simulink model "gyroboy_ext"  (R2019a)
settings: Solver=FixedStepAuto  StartTime=0.0  StopTime=inf  FixedStep=Ts  RelTol=1e-3  EnableMultiTasking=on
PreLoadFcn:
  | config
  | preload
  | HW=1;
InitFcn:
  | plant
  | control
undefined symbols (not defined in the file): A1, A2, B1, B2, C1, C2, D, D1, D2, DiscIntNeverNeededParam, fw, g, h, Jm, Jw, K, K_PWM, M, Psi0, R, Ts, W, X, Y, Z
libraries: sm_lib x16, nesl_utility x10, legoev3lib x9, simulink_extras x3, simulink x3, discretizing x1
settings Model: SimulationMode=external  ExtModeTrigDuration=20000  Creator=roslovetspv  LastModifiedBy=Pavel Roslovets
settings SolverCC: ZeroCrossAlgorithm=Adaptive  PositivePriorityOrder=on
settings OptimizationCC: MaxStackSize=64
settings DebuggingCC: ParameterTunabilityLossMsg=error  PregeneratedLibrarySubsystemCodeDiagnostic=none  ArithmeticOperatorsInVariantConditions=warning
settings HardwareCC: ProdBitPerPointer=32  ProdBitPerSizeT=32  ProdBitPerPtrDiffT=32  ProdLargestAtomicInteger=Long  ProdWordSize=32  ProdHWDeviceType=ARM Compatible->ARM 9
settings SFSimCC: SimUseLocalCustomCode=off  MATLABDynamicMemAlloc=off
settings RTWCC: SystemTargetFile=ert.tlc  HardwareBoard=LEGO MINDSTORMS EV3  TLCOptions="-aInlineSetEventsForThisBaseRateFcn=TLC_FALSE -aSuppressMultiTaskScheduler=TLC_FALSE  -aRateBasedStepFcn=0"  TemplateMakefile=ert_default_tmf  GenerateReport=on  RTWUseLocalCustomCode=off  Toolchain=Sourcery G++ Lite v2009q3  IncludeHyperlinkInReport=on  LaunchReport=on  GenerateTraceInfo=on  GenerateTraceReport=on  GenerateTraceReportSl=on  GenerateTraceReportSf=on  GenerateTraceReportEml=on
settings CodeAppCC: ForceParamTrailComments=on  IgnoreCustomStorageClasses=off  OperatorAnnotations=on  SimulinkDataObjDesc=on  SFDataObjDesc=on  MATLABFcnDesc=on  InsertBlockDesc=on  StateflowObjectComments=on  MATLABSourceComments=on
settings ERTTargetCC: MultiwordLength=2048  SupportContinuousTime=on  SupportVariableSizeSignals=on
settings ExplorerConfigSet: InternalSimMechanicsExplorerSettings="<ExplorerConfiguration><canonicalview>default</canonicalview><AnimationSetting><BasePlaybackSpeed>1.0</BasePlaybackSpeed><PlaybackSpeedFactor>1.0</PlaybackSpeedFactor></AnimationSetting><TilePanel><TileInfo><Tiles Columns=\"1\" Count=\"1\" Rows=\"1\"><Column Weight=\"1\"/><Row Weight=\"1\"/><Tile Height=\"1\" Width=\"1\" X=\"0\" Y=\"0\"/></Tiles></TileInfo><SceneInfo><SceneViewer><BGColor><R>1</R><G>1</G><B>1</B></BGColor><Camera><DoPerspective>off</DoPerspective><Position><X>0.737677845990044934</X><Y>-0.67856704951033231</Y><Z>0.394310698325195552</Z></Position><Center><X>0.13835347465754938</X><Y>0.0549599908195436276</Y><Z>0.0737668182840573866</Z></Center><Up><X>-0.28491224059991338</X><Y>0.178745032231141465</Y><Z>0.941740531467678998</Z></Up><ViewLimDist>1</ViewLimDist><YLim>0.238341914277370809</YLim><XLim>0.445475675236847168</XLim></Camera></SceneViewer></SceneInfo></TilePanel><MechEditorPanel><Cameras/><GfxPanelCameraMap/><VideoCreator><PlaybackSpeedRatio>1.0</PlaybackSpeedRatio><FrameRate>30</FrameRate><VideoFormat>Motion JPEG AVI</VideoFormat><FrameSize>auto</FrameSize></VideoCreator></MechEditorPanel></ExplorerConfiguration>"

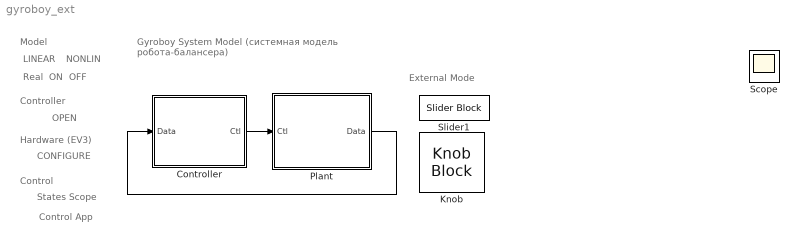
== system gyroboy_ext ==
  note: External Mode
  note: Control
  note: States Scope
  note: OPEN
  note: Controller
  note: Hardware (EV3)
  note: Model
  note: Real
  note: Gyroboy System Model
      | (системная модель робота-балансера)
  note: ON
  note: OFF
  note: CONFIGURE
  note: LINEAR
  note: NONLIN
  note: Control App
  Controller : Subsystem
      mask Display: image('img/brain.png')
  Knob : KnobBlock  ScaleMin=-10  ScaleMax=10  TickInterval=1
  Plant : Subsystem  Variant=on  VariantControl=Variant1
      mask Display:
      | if evalin('base','HW')
      |     image('img/gyroboy.png')
      | elseif evalin('base','MB')
      |     image('img/multibody.png')
      | else
      |     image('img/math.png')
      | end
  Slider1 : SliderBlock  ScaleMin=-10  ScaleMax=10  TickInterval=1
  Scope : Scope
  wires:
  Controller/1(Ctl) -> Plant/1("Ctl ")
  Plant/1(" Data") -> Controller/1(Data)

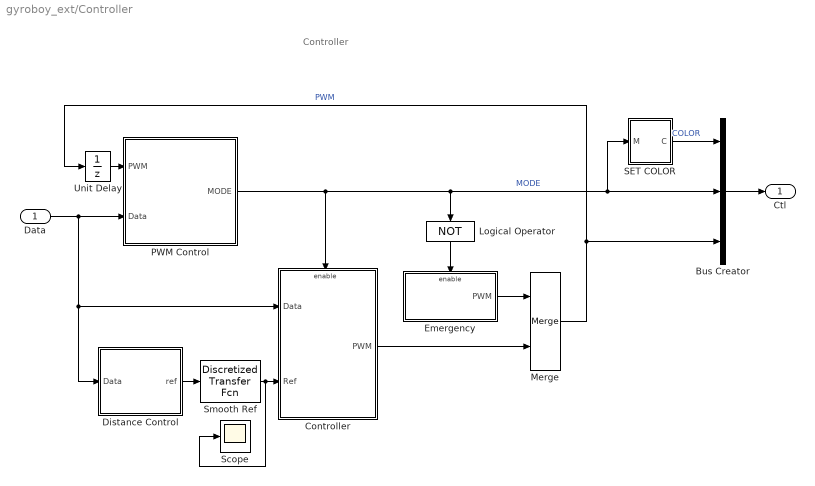
== system gyroboy_ext/Controller ==
  note: Controller
  Data : Inport
  Bus Creator : BusCreator  Inputs=3
  Controller : Subsystem  TreatAsAtomicUnit=on
      mask Display: disp('ON')
  Distance Control : Stateflow chart  TreatAsAtomicUnit=on
  Emergency : Subsystem  TreatAsAtomicUnit=on
      mask Display: disp('OFF')
  Logical Operator : Logic  Operator=NOT  AllPortsSameDT=off  OutDataTypeStr=boolean
  Merge : Merge
  PWM Control : Stateflow chart  TreatAsAtomicUnit=on
  SET COLOR : MATLAB Function  TreatAsAtomicUnit=on
  Scope : Scope
  Smooth Ref : discretizing/Discretized Transfer Fcn  Numerator=[1]  Denominator=[0.7 1]  AbsTol=auto  SampleTime=Ts  method=zoh  Wc=1
      settings: SourceProductName=Simulink  SourceProductBaseCode=SL
  Unit Delay : UnitDelay  SampleTime=-1  HasFrameUpgradeWarning=on
  Ctl : Outport
  wires:
  Merge/1 -> Unit Delay/1, Bus Creator/3  "PWM"
  PWM Control/1(MODE) -> Logical Operator/1, Bus Creator/2, SET COLOR/1(M), Controller/Enable  "MODE"
  Data/1 -> PWM Control/2(Data), Distance Control/1(Data), Controller/1(Data)
  Controller/1(PWM) -> Merge/2
  Emergency/1(PWM) -> Merge/1
  Unit Delay/1 -> PWM Control/1(PWM)
  Logical Operator/1 -> Emergency/Enable
  Bus Creator/1 -> Ctl/1
  SET COLOR/1(C) -> Bus Creator/1  "COLOR"
  Distance Control/1(ref) -> Smooth Ref/1
  Smooth Ref/1 -> Scope/1, Controller/2(Ref)

== system gyroboy_ext/Plant ==
  "Ctl " : Inport
  EV3 : Subsystem  VariantControl=HW==1
  Model : Subsystem  VariantControl=(default)
  " Data" : Outport

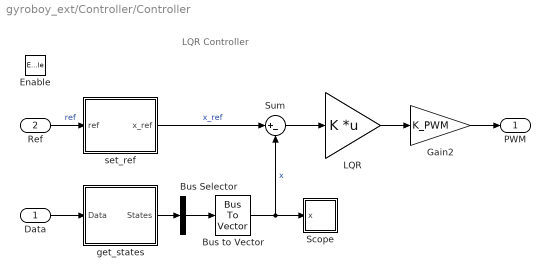
== system gyroboy_ext/Controller/Controller ==
  note: LQR Controller
  Data : Inport
  Ref : Inport  Port=2
  Enable : EnablePort  StatesWhenEnabling=reset
  Bus Selector : BusSelector  OutputSignals=theta_int,theta,psi,theta_dot,psi_dot,phi,phi_dot  OutputAsBus=on
  Bus to Vector : BusToVector
  Gain2 : Gain  Gain=K_PWM
  LQR : Gain  Gain=K  Multiplication=Matrix(K*u)
  Scope : Subsystem
  Sum : Sum  Inputs=|+-
  get_states : Subsystem
  set_ref : Subsystem
  PWM : Outport
  wires:
  Data/1 -> get_states/1(Data)
  Sum/1 -> LQR/1
  Bus Selector/1 -> Bus to Vector/1
  get_states/1(States) -> Bus Selector/1
  LQR/1 -> Gain2/1
  Bus to Vector/1 -> Sum/2, Scope/1(x)  "x"
  Ref/1 -> set_ref/1(ref)  "ref"
  Gain2/1 -> PWM/1
  set_ref/1(x_ref) -> Sum/1  "x_ref"

== system gyroboy_ext/Controller/Distance Control/Normal ==
  Data : Inport  OutDataTypeStr=Bus: Data
  Action Port : ActionPort
      settings: CopyFcn=Stateflow.SLINSF.SimulinkMan.removeBlockPreDeleteFcn  PreDeleteFcn=Stateflow.SLINSF.SimulinkMan.unsafePredeleteFcn
  Bus Selector2 : BusSelector  OutputSignals=udp
  Demux : Demux  Outputs=2
  Gain : Gain  Gain=0.75
  Gain1 : Gain  Gain=0.2
  Mux : Mux  Inputs=2
  ref : Outport  PortDimensions=2
  wires:
  Gain1/1 -> Mux/2
  Mux/1 -> ref/1  "ref"
  Gain/1 -> Mux/1
  Demux/1 -> Gain/1  "Vel"
  Demux/2 -> Gain1/1  "Turn"
  Data/1 -> Bus Selector2/1
  Bus Selector2/1 -> Demux/1  "<udp>"

== system gyroboy_ext/Controller/Distance Control/STOP ==
  Data : Inport  OutDataTypeStr=Bus: Data
  Action Port : ActionPort
      settings: CopyFcn=Stateflow.SLINSF.SimulinkMan.removeBlockPreDeleteFcn  PreDeleteFcn=Stateflow.SLINSF.SimulinkMan.unsafePredeleteFcn
  Constant : Constant  Value=[0 0]
  Terminator : Terminator
  ref : Outport  PortDimensions=2
  wires:
  Data/1 -> Terminator/1
  Constant/1 -> ref/1

== system gyroboy_ext/Controller/Emergency ==
  Enable : EnablePort  StatesWhenEnabling=reset
  Constant : Constant  Value=[0 0]
  PWM : Outport
  wires:
  Constant/1 -> PWM/1

== system gyroboy_ext/Controller/PWM Control/On.check ==
  PWM : Inport  OutDataTypeStr=double  PortDimensions=2
  f : TriggerPort  TriggerType=function-call  VariantControl=(inherit)
      settings: CopyFcn=Stateflow.SLINSF.SimulinkMan.removeBlockPreDeleteFcn  PreDeleteFcn=Stateflow.SLINSF.SimulinkMan.unsafePredeleteFcn
  Abs : Abs
  Compare To Constant : simulink/Logic and Bit Operations/Compare To Constant  relop=<  const=200  OutDataTypeStr=boolean
  Sum of Elements : Sum  Inputs=+
  OK : Outport  PortDimensions=1
  wires:
  PWM/1 -> Abs/1
  Abs/1 -> Sum of Elements/1
  Sum of Elements/1 -> Compare To Constant/1
  Compare To Constant/1 -> OK/1

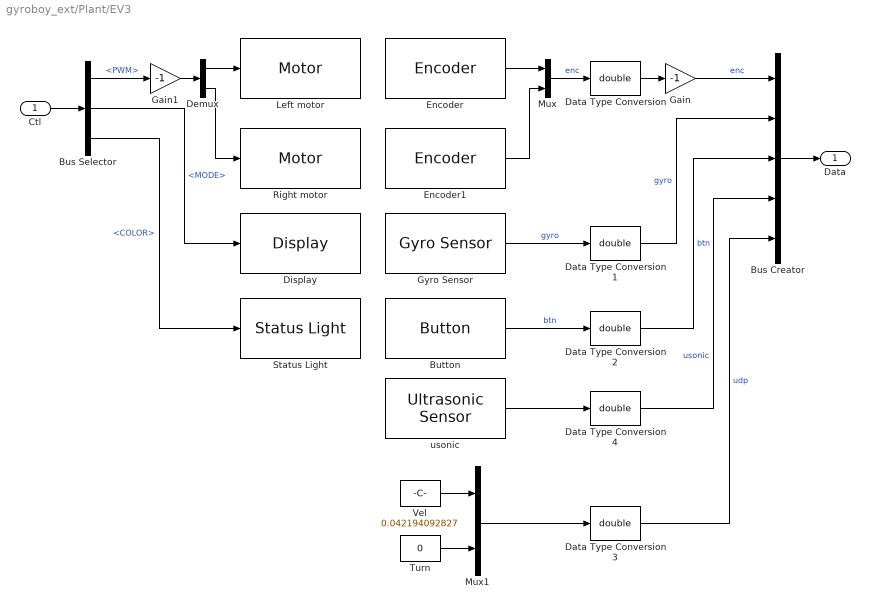
== system gyroboy_ext/Plant/EV3 ==
  Ctl : Inport
  Bus Creator : BusCreator  Inputs=5
  Bus Selector : BusSelector  OutputSignals=PWM,MODE,COLOR
  Button : legoev3lib/Button  buttonType=Up  sampleTime=Ts
      settings: SourceProductName=Simulink Support Package for LEGO MINDSTORMS EV3 Hardware  SourceProductBaseCode=LEGOEV3
  Data Type Conversion{,1..4} (5 alike) : DataTypeConversion  OutDataTypeStr=double
  Demux : Demux  Outputs=2
  Display : legoev3lib/Display  slcdStr=RUNNING  slcdLine=1  slcdFormat=Decimal
      settings: SourceProductName=Simulink Support Package for LEGO MINDSTORMS EV3 Hardware  SourceProductBaseCode=LEGOEV3
  Encoder : legoev3lib/Encoder  portNumber=D  opMode=No reset  sampleTime=Ts
      settings: SourceProductName=Simulink Support Package for LEGO MINDSTORMS EV3 Hardware  SourceProductBaseCode=LEGOEV3
  Encoder1 : legoev3lib/Encoder  portNumber=A  opMode=No reset  sampleTime=Ts
      settings: SourceProductName=Simulink Support Package for LEGO MINDSTORMS EV3 Hardware  SourceProductBaseCode=LEGOEV3
  Gain : Gain  Gain=-1
  Gain1 : Gain  Gain=-1
  Gyro Sensor : legoev3lib/Gyro Sensor  portNumber=2  sampleTime=Ts
      settings: SourceProductName=Simulink Support Package for LEGO MINDSTORMS EV3 Hardware  SourceProductBaseCode=LEGOEV3
  Left motor : legoev3lib/Motor  sportNumber=D  sstopAction=Brake
  Mux : Mux  Inputs=2
  Mux1 : Mux  Inputs=2
  Right motor : legoev3lib/Motor  sportNumber=A  sstopAction=Brake
  Status Light : legoev3lib/Status Light
      settings: SourceProductName=Simulink Support Package for LEGO MINDSTORMS EV3 Hardware  SourceProductBaseCode=LEGOEV3
  Turn : Constant  Value=0
  Vel : Constant  Value=0.042194092827
  usonic : legoev3lib/Ultrasonic Sensor  PortNumber=4  sampleTime=Ts
      settings: SourceProductName=Simulink Support Package for LEGO MINDSTORMS EV3 Hardware  SourceProductBaseCode=LEGOEV3
  Data : Outport
  wires:
  Ctl/1 -> Bus Selector/1
  Encoder/1 -> Mux/1
  Encoder1/1 -> Mux/2
  Gyro Sensor/1 -> Data Type Conversion1/1  "gyro"
  Bus Selector/1 -> Gain1/1  "<PWM>"
  Mux/1 -> Data Type Conversion/1  "enc"
  Bus Creator/1 -> Data/1
  Demux/1 -> Left motor/1
  Demux/2 -> Right motor/1
  Data Type Conversion/1 -> Gain/1
  Data Type Conversion1/1 -> Bus Creator/2  "gyro"
  Gain/1 -> Bus Creator/1  "enc"
  Gain1/1 -> Demux/1
  Bus Selector/2 -> Display/1  "<MODE>"
  Button/1 -> Data Type Conversion2/1  "btn"
  Data Type Conversion2/1 -> Bus Creator/3  "btn"
  Bus Selector/3 -> Status Light/1  "<COLOR>"
  Data Type Conversion3/1 -> Bus Creator/5  "udp"
  usonic/1 -> Data Type Conversion4/1
  Data Type Conversion4/1 -> Bus Creator/4  "usonic"
  Vel/1 -> Mux1/1
  Turn/1 -> Mux1/2
  Mux1/1 -> Data Type Conversion3/1

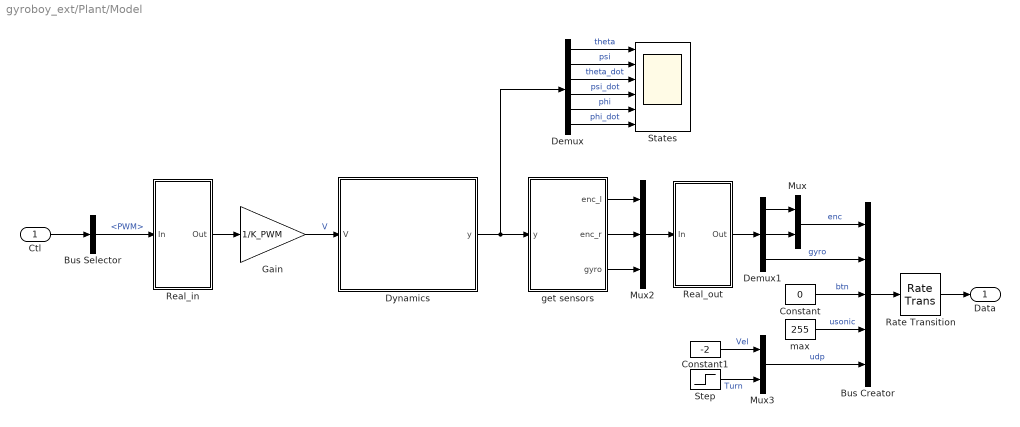
== system gyroboy_ext/Plant/Model ==
  Ctl : Inport
  Bus Creator : BusCreator  Inputs=5
  Bus Selector : BusSelector  OutputSignals=PWM
  Constant : Constant  Value=0
  Constant1 : Constant  Value=-2
  Demux : Demux  Outputs=6
  Demux1 : Demux  Outputs=3
  Dynamics : Subsystem  Variant=on  VariantControl=Variant1
  Gain : Gain  Gain=1/K_PWM
  Mux : Mux  Inputs=2
  Mux2 : Mux  Inputs=3
  Mux3 : Mux  Inputs=2
  Rate Transition : RateTransition  OutPortSampleTime=Ts
  Real_in : Subsystem  Variant=on  VariantControl=Variant1
  Real_out : Subsystem  Variant=on  VariantControl=Variant1
  States : Scope  NumInputPorts=6
  Step : Step  Time=3  Before=1  After=0  SampleTime=0
  get sensors : MATLAB Function  TreatAsAtomicUnit=on
  max : Constant  Value=255
  Data : Outport
  wires:
  Real_in/1(" Out") -> Gain/1
  Ctl/1 -> Bus Selector/1
  Mux2/1 -> Real_out/1("In ")
  get sensors/3(gyro) -> Mux2/3
  Real_out/1(" Out") -> Demux1/1
  Demux/4 -> States/4  "psi_dot"
  Demux/6 -> States/6  "phi_dot"
  Demux/5 -> States/5  "phi"
  Bus Creator/1 -> Rate Transition/1
  Demux1/1 -> Mux/1
  Demux1/2 -> Mux/2
  Demux1/3 -> Bus Creator/2  "gyro"
  Demux/2 -> States/2  "psi"
  Demux/3 -> States/3  "theta_dot"
  Demux/1 -> States/1  "theta"
  Bus Selector/1 -> Real_in/1(In)  "<PWM>"
  get sensors/1(enc_l) -> Mux2/1
  get sensors/2(enc_r) -> Mux2/2
  Mux/1 -> Bus Creator/1  "enc"
  Rate Transition/1 -> Data/1
  Constant/1 -> Bus Creator/3  "btn"
  Constant1/1 -> Mux3/1  "Vel"
  Step/1 -> Mux3/2  "Turn"
  Mux3/1 -> Bus Creator/5  "udp"
  Gain/1 -> Dynamics/1("V ")  "V"
  Dynamics/1(" y") -> Demux/1, get sensors/1(y)
  max/1 -> Bus Creator/4  "usonic"

== system gyroboy_ext/Controller/Controller/Scope ==
  x : Inport
  Demux : Demux  Outputs=7
  Scope : Scope  NumInputPorts=7
  wires:
  Demux/7 -> Scope/7  "phi_dot"
  Demux/5 -> Scope/5  "psi_dot"
  Demux/3 -> Scope/3  "psi"
  Demux/6 -> Scope/6  "phi"
  Demux/2 -> Scope/2  "theta"
  Demux/1 -> Scope/1  "theta_int"
  Demux/4 -> Scope/4  "theta_dot"
  x/1 -> Demux/1

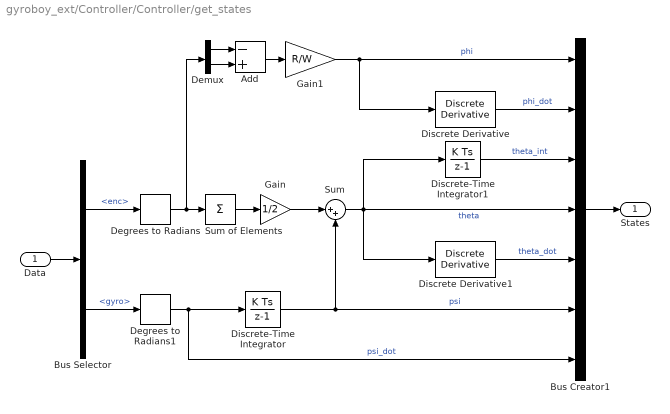
== system gyroboy_ext/Controller/Controller/get_states ==
  Data : Inport
  Add : Sum  Inputs=-+
  Bus Creator1 : BusCreator  Inputs=7
  Bus Selector : BusSelector  OutputSignals=enc,gyro
  Degrees to Radians : simulink_extras/Transformations/Degrees to Radians
  Degrees to Radians1 : simulink_extras/Transformations/Degrees to Radians
  Demux : Demux  Outputs=2
  Discrete Derivative : simulink/Discrete/Discrete Derivative  gainval=1.0  ICPrevScaledInput=0.0  OutMin=[]  OutMax=[]  OutDataType=fixdt(1, 16)  OutScaling=2^-10  DoSatur=off
  Discrete Derivative1 : simulink/Discrete/Discrete Derivative  gainval=1.0  ICPrevScaledInput=0.0  OutMin=[]  OutMax=[]  OutDataType=fixdt(1, 16)  OutScaling=2^-10  DoSatur=off
  Discrete-Time Integrator : DiscreteIntegrator  SampleTime=-1  ICPrevOutput=DiscIntNeverNeededParam  ICPrevScaledInput=DiscIntNeverNeededParam
  Discrete-Time Integrator1 : DiscreteIntegrator  SampleTime=-1  ICPrevOutput=DiscIntNeverNeededParam  ICPrevScaledInput=DiscIntNeverNeededParam
  Gain : Gain  Gain=1/2
  Gain1 : Gain  Gain=R/W
  Sum : Sum  Inputs=|++
  Sum of Elements : Sum  Inputs=+
  States : Outport
  wires:
  Gain/1 -> Sum/1
  Degrees to Radians/1 -> Demux/1, Sum of Elements/1
  Data/1 -> Bus Selector/1
  Bus Selector/1 -> Degrees to Radians/1  "<enc>"
  Sum/1 -> Discrete-Time Integrator1/1, Discrete Derivative1/1, Bus Creator1/4  "theta"
  Bus Creator1/1 -> States/1
  Sum of Elements/1 -> Gain/1
  Degrees to Radians1/1 -> Discrete-Time Integrator/1, Bus Creator1/7  "psi_dot"
  Bus Selector/2 -> Degrees to Radians1/1  "<gyro>"
  Demux/1 -> Add/1
  Demux/2 -> Add/2
  Add/1 -> Gain1/1
  Gain1/1 -> Discrete Derivative/1, Bus Creator1/1  "phi"
  Discrete Derivative/1 -> Bus Creator1/2  "phi_dot"
  Discrete Derivative1/1 -> Bus Creator1/5  "theta_dot"
  Discrete-Time Integrator/1 -> Sum/2, Bus Creator1/6  "psi"
  Discrete-Time Integrator1/1 -> Bus Creator1/3  "theta_int"

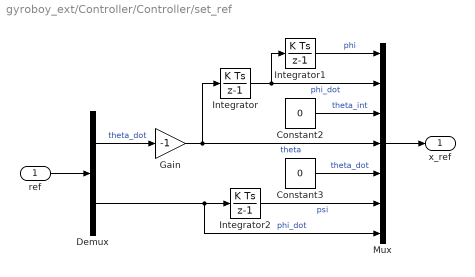
== system gyroboy_ext/Controller/Controller/set_ref ==
  ref : Inport
  Constant2 : Constant  Value=0
  Constant3 : Constant  Value=0
  Demux : Demux  Outputs=2
  Gain : Gain  Gain=-1
  Integrator : DiscreteIntegrator  SampleTime=Ts  ICPrevOutput=DiscIntNeverNeededParam  ICPrevScaledInput=DiscIntNeverNeededParam  mask(DiscretizedDiscreteIntegrator){}
      mask init:
      | %zoh
  Integrator1 : DiscreteIntegrator  SampleTime=Ts  ICPrevOutput=DiscIntNeverNeededParam  ICPrevScaledInput=DiscIntNeverNeededParam  mask(DiscretizedDiscreteIntegrator){}
      mask init:
      | %zoh
  Integrator2 : DiscreteIntegrator  SampleTime=Ts  ICPrevOutput=DiscIntNeverNeededParam  ICPrevScaledInput=DiscIntNeverNeededParam  mask(DiscretizedDiscreteIntegrator){}
      mask init:
      | %zoh
  Mux : Mux  Inputs=7
  x_ref : Outport
  wires:
  Constant2/1 -> Mux/3  "theta_int"
  Constant3/1 -> Mux/5  "theta_dot"
  Mux/1 -> x_ref/1
  Integrator/1 -> Mux/2, Integrator1/1  "phi_dot"
  Demux/2 -> Mux/7, Integrator2/1  "phi_dot"
  Integrator2/1 -> Mux/6  "psi"
  Integrator1/1 -> Mux/1  "phi"
  Demux/1 -> Gain/1  "theta_dot"
  ref/1 -> Demux/1
  Gain/1 -> Integrator/1, Mux/4  "theta"

== system gyroboy_ext/Plant/Model/Dynamics ==
  "V " : Inport
  Multibody (nonlinear) : Subsystem  VariantControl=MB == 1
  State-space (linear) : Subsystem  VariantControl=(default)
  " y" : Outport

== system gyroboy_ext/Plant/Model/Real_in ==
  In : Inport
  Ideal_in : Subsystem  VariantControl=(default)
  Real_in : Subsystem  VariantControl=real_model == 1
  " Out" : Outport

== system gyroboy_ext/Plant/Model/Real_out ==
  "In " : Inport
  Ideal_out : Subsystem  VariantControl=(default)
  Real_out : Subsystem  VariantControl=real_model == 1
  " Out" : Outport

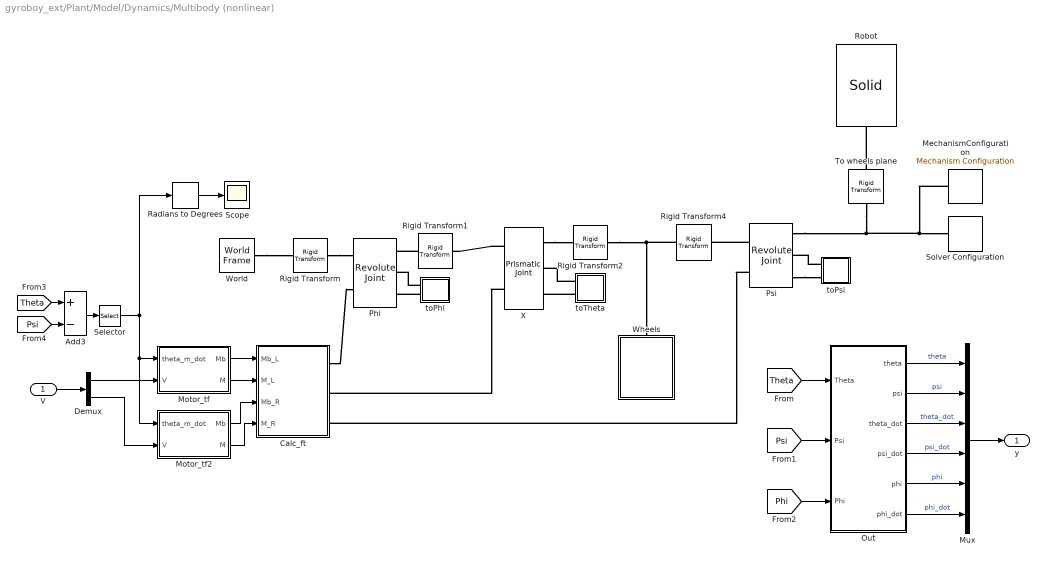
== system gyroboy_ext/Plant/Model/Dynamics/Multibody (nonlinear) ==
  V : Inport
  Add3 : Sum  Inputs=+-
  Calc_ft : Subsystem
  Demux : Demux  Outputs=2
  MechanismConfiguration : sm_lib/Utilities/Mechanism Configuration  UniformGravity=Constant  GravityVector=[0 0 -g]  GravityUnits=m/s^2  LinearizationDelta=0.00001
  Motor_tf : Subsystem  mask{Kt=0.0209, Rm=1, b=0.0113, Km=0, Tm=0}
  Motor_tf2 : Subsystem  mask{Kt=0.0209, Rm=1, b=0.0113, Km=0, Tm=0}
  Mux : Mux  Inputs=6
  Out : Subsystem
  Phi : sm_lib/Joints/Revolute Joint  SenseConstraintForce=off  SenseConstraintForceX=off  SenseConstraintForceY=off  SenseConstraintForceZ=off  SenseConstraintTorque=off  SenseConstraintTorqueX=off  SenseConstraintTorqueY=off  SenseConstraintTorqueZ=off  SenseTotalForce=off  SenseTotalForceX=off  SenseTotalForceY=off  SenseTotalForceZ=off  SenseTotalTorque=off  SenseTotalTorqueX=off  SenseTotalTorqueY=off  SenseTotalTorqueZ=off  CompositeWrenchDir=FollowerOnBase  CompositeWrenchFrame=BaseFrame  EquilibriumPosition=0  EquilibriumPositionUnits=deg  SpringStiffness=0  SpringStiffnessUnits=N*m/deg  DampingCoefficient=W^2/R^2/2*(0.0113+fw)  DampingCoefficientUnits=N*m/(rad/s)  TorqueActuationMode=InputTorque  MotionActuationMode=ComputedMotion  SensePosition=on  SenseVelocity=on  SenseAcceleration=off  SenseTorqueForce=off  SenseLowerLimitTorqueForce=off  SenseUpperLimitTorqueForce=off  LowerLimitSpecify=off  LowerLimitBound=-90  LowerLimitBoundUnits=deg  LowerLimitStiffness=1e4  LowerLimitStiffnessUnits=N*m/deg  LowerLimitDamping=10  LowerLimitDampingUnits=N*m/(deg/s)  LowerLimitTransitionRegionWidth=0.1  LowerLimitTransitionRegionWidthUnits=deg  UpperLimitSpecify=off  UpperLimitBound=90  UpperLimitBoundUnits=deg  UpperLimitStiffness=1e4  UpperLimitStiffnessUnits=N*m/deg  UpperLimitDamping=10  UpperLimitDampingUnits=N*m/(deg/s)  UpperLimitTransitionRegionWidth=0.1  UpperLimitTransitionRegionWidthUnits=deg  PositionTargetSpecify=off  PositionTargetPriority=High  PositionTargetValue=0  PositionTargetValueUnits=deg  VelocityTargetSpecify=off  VelocityTargetPriority=High  VelocityTargetValue=0  VelocityTargetValueUnits=deg/s
  Psi : sm_lib/Joints/Revolute Joint  SenseConstraintForce=off  SenseConstraintForceX=off  SenseConstraintForceY=off  SenseConstraintForceZ=off  SenseConstraintTorque=off  SenseConstraintTorqueX=off  SenseConstraintTorqueY=off  SenseConstraintTorqueZ=off  SenseTotalForce=off  SenseTotalForceX=off  SenseTotalForceY=off  SenseTotalForceZ=off  SenseTotalTorque=off  SenseTotalTorqueX=off  SenseTotalTorqueY=off  SenseTotalTorqueZ=off  CompositeWrenchDir=FollowerOnBase  CompositeWrenchFrame=BaseFrame  EquilibriumPosition=0  EquilibriumPositionUnits=deg  SpringStiffness=0  SpringStiffnessUnits=N*m/deg  DampingCoefficient=0  DampingCoefficientUnits=N*m/(deg/s)  TorqueActuationMode=InputTorque  MotionActuationMode=ComputedMotion  SensePosition=on  SenseVelocity=on  SenseAcceleration=off  SenseTorqueForce=off  SenseLowerLimitTorqueForce=off  SenseUpperLimitTorqueForce=off  LowerLimitSpecify=off  LowerLimitBound=-90  LowerLimitBoundUnits=deg  LowerLimitStiffness=1e4  LowerLimitStiffnessUnits=N*m/deg  LowerLimitDamping=10  LowerLimitDampingUnits=N*m/(deg/s)  LowerLimitTransitionRegionWidth=0.1  LowerLimitTransitionRegionWidthUnits=deg  UpperLimitSpecify=off  UpperLimitBound=90  UpperLimitBoundUnits=deg  UpperLimitStiffness=1e4  UpperLimitStiffnessUnits=N*m/deg  UpperLimitDamping=10  UpperLimitDampingUnits=N*m/(deg/s)  UpperLimitTransitionRegionWidth=0.1  UpperLimitTransitionRegionWidthUnits=deg  PositionTargetSpecify=on  PositionTargetPriority=High  PositionTargetValue=Psi0  PositionTargetValueUnits=rad  VelocityTargetSpecify=off  VelocityTargetPriority=High  VelocityTargetValue=1  VelocityTargetValueUnits=deg/s
  Radians to Degrees : simulink_extras/Transformations/Radians to Degrees
  Rigid Transform : sm_lib/Frames and Transforms/Rigid Transform  TranslationMethod=Cartesian  TranslationStandardOffset=0  TranslationLengthUnit=m  TranslationStandardAxis=+Z  TranslationCartesianOffset=[0 0 R]  TranslationROffset=0  TranslationROffsetUnits=m  TranslationZOffset=0  TranslationZOffsetUnits=m  TranslationThetaOffset=0  TranslationThetaOffsetUnits=deg  RotationMethod=None  RotationAngleUnits=deg  RotationStandardAxis=+Z  RotationAngle=0.0  RotationArbitraryAxis=[0 0 1]  FollAlignAxisA=+X  BaseAlignAxisA=+Y  FollAlignAxisB=+Y  BaseAlignAxisB=+Z  RotationSequenceAxes=FollowerAxes  RotationSequence=XYX  RotationSequenceAngles=[0 0 0]  RotationSequenceAnglesUnits=deg  RotationMatrix=[1 0 0; 0 1 0; 0 0 1]
  Rigid Transform1 : sm_lib/Frames and Transforms/Rigid Transform  TranslationMethod=None  TranslationStandardOffset=0  TranslationLengthUnit=m  TranslationStandardAxis=+Z  TranslationCartesianOffset=[0 0 0]  TranslationROffset=0  TranslationROffsetUnits=m  TranslationZOffset=0  TranslationZOffsetUnits=m  TranslationThetaOffset=0  TranslationThetaOffsetUnits=deg  RotationMethod=StandardAxis  RotationAngleUnits=deg  RotationStandardAxis=+Y  RotationAngle=90  RotationArbitraryAxis=[0 0 1]  FollAlignAxisA=+X  BaseAlignAxisA=+Y  FollAlignAxisB=+Y  BaseAlignAxisB=+Z  RotationSequenceAxes=FollowerAxes  RotationSequence=XYX  RotationSequenceAngles=[0 0 0]  RotationSequenceAnglesUnits=deg  RotationMatrix=[1 0 0; 0 1 0; 0 0 1]
  Rigid Transform2 : sm_lib/Frames and Transforms/Rigid Transform  TranslationMethod=None  TranslationStandardOffset=0  TranslationLengthUnit=m  TranslationStandardAxis=+Z  TranslationCartesianOffset=[0 0 0]  TranslationROffset=0  TranslationROffsetUnits=m  TranslationZOffset=0  TranslationZOffsetUnits=m  TranslationThetaOffset=0  TranslationThetaOffsetUnits=deg  RotationMethod=StandardAxis  RotationAngleUnits=deg  RotationStandardAxis=+Y  RotationAngle=90  RotationArbitraryAxis=[0 0 1]  FollAlignAxisA=+X  BaseAlignAxisA=+Y  FollAlignAxisB=+Y  BaseAlignAxisB=+Z  RotationSequenceAxes=FollowerAxes  RotationSequence=XYX  RotationSequenceAngles=[0 0 0]  RotationSequenceAnglesUnits=deg  RotationMatrix=[1 0 0; 0 1 0; 0 0 1]
  Rigid Transform4 : sm_lib/Frames and Transforms/Rigid Transform  TranslationMethod=None  TranslationStandardOffset=0  TranslationLengthUnit=m  TranslationStandardAxis=+Z  TranslationCartesianOffset=[0 -W/2 0]  TranslationROffset=0  TranslationROffsetUnits=m  TranslationZOffset=0  TranslationZOffsetUnits=m  TranslationThetaOffset=0  TranslationThetaOffsetUnits=deg  RotationMethod=StandardAxis  RotationAngleUnits=deg  RotationStandardAxis=-X  RotationAngle=90  RotationArbitraryAxis=[0 0 1]  FollAlignAxisA=+X  BaseAlignAxisA=+Y  FollAlignAxisB=+Y  BaseAlignAxisB=+Z  RotationSequenceAxes=FollowerAxes  RotationSequence=XYX  RotationSequenceAngles=[0 0 0]  RotationSequenceAnglesUnits=deg  RotationMatrix=[1 0 0; 0 1 0; 0 0 1]
  Robot : sm_lib/Body Elements/Solid  InertiaType=CalculateFromGeometry  Mass=M  MassUnits=kg  CenterOfMass=[0 0 0]  CenterOfMassUnits=m  MomentsOfInertia=[1 1 1]  MomentsOfInertiaUnits=kg*m^2  ProductsOfInertia=[0 0 0]  ProductsOfInertiaUnits=kg*m^2  BasedOnType=Mass  Density=1000  DensityUnits=kg/(m^3)  DoExposeReferenceFrame=on  SerializedFrames=<Frames/>  GraphicType=FromGeometry  MarkerShape=Sphere  MarkerSize=10  GraphicVisPropType=SimpleVisualProperties  GraphicDiffuseColor=[0.0 1.0 0.4]  GraphicSpecularColor=[0.5 0.5 0.5 1.0]  GraphicAmbientColor=[0.15 0.15 0.15 1.0]  GraphicEmissiveColor=[0.0 0.0 0.0 1.0]  GraphicShininess=75  GraphicOpacity=1.0  GeometryShape=Brick  RectangleSize=[1 1]  RectangleSizeUnits=m  BrickDimensions=[D h W]  BrickDimensionUnits=m  CylinderRadius=1  CylinderRadiusUnits=m  CylinderLength=1  CylinderLengthUnits=m  SphereRadius=1  SphereRadiusUnits=m  EllipsoidRadii=[1 1 1]  EllipsoidRadiiUnits=m  ExtrusionCrossSection=[1 1; -1 1; -1 -1; 1 -1]  ExtrusionCrossSectionUnits=m  ExtrusionLength=1  ExtrusionLengthUnits=m  PolygonNumSides=3  PolygonOuterRadius=1  PolygonOuterRadiusUnits=m  ExtGeomFileType=STEP  ExtGeomFileUnits=m  RevolutionCrossSection=[1 1; 1 -1; 2 -1; 2 1]  RevolutionCrossSectionUnits=m  RevolutionExtent=Full  RevolutionAngle=180  RevolutionAngleUnits=deg
  Scope : Scope
  Selector : Selector  InputPortWidth=2  IndexOptions=Index vector (dialog)  Indices=2  OutputSizes=1
  Solver Configuration : nesl_utility/Solver Configuration  PhysicalDomain=network_engine_domain  SubClassName=solver  LeftPortType=input  RightPortType=generic  Tones=[]  Harmonics=[]  SimulateNoise=off  Profile=off  UseLocalSampling=off  EnableSwitchedLinearOptims=on  FrequencyDomain=off  UseCCode=off  RelTol=0.001  AbsTol=1e-06  MinStep=1e-09  ToWorkspace=off  RevertToSquareIcSolve=off  NumHomotopyIterations=100  PhasorMode=off  PhasorModeNumHarmonics=1  DoDC=off  ResidualTolerance=1e-09  UseLocalSolver=off  LocalSolverChoice=NE_TRAPEZOIDAL_ADVANCER  LocalSolverSampleTime=0.001  DoFixedCost=off  MaxNonlinIter=3  MaxModeIter=2  LinearAlgebra=Sparse  EquationFormulation=NE_TIME_EF  DelaysMemoryBudget=1024  AutomaticFiltering=on  FilteringTimeConstant=1e-6  PartitionStorageMethod=AS_NEEDED  PartitionMemoryBudget=1024  PartitionMethod=FAST
  To wheels plane : sm_lib/Frames and Transforms/Rigid Transform  TranslationMethod=Cartesian  TranslationStandardOffset=0  TranslationLengthUnit=m  TranslationStandardAxis=+Z  TranslationCartesianOffset=[0 h/2 0]  TranslationROffset=0  TranslationROffsetUnits=m  TranslationZOffset=0  TranslationZOffsetUnits=m  TranslationThetaOffset=0  TranslationThetaOffsetUnits=deg  RotationMethod=None  RotationAngleUnits=deg  RotationStandardAxis=+Z  RotationAngle=0.0  RotationArbitraryAxis=[0 0 1]  FollAlignAxisA=+X  BaseAlignAxisA=+Y  FollAlignAxisB=+Y  BaseAlignAxisB=+Z  RotationSequenceAxes=FollowerAxes  RotationSequence=XYX  RotationSequenceAngles=[0 0 0]  RotationSequenceAnglesUnits=deg  RotationMatrix=[1 0 0; 0 1 0; 0 0 1]
  Wheels : Subsystem
      mask Display:
      | plot(sin(0:0.01:10), cos(0:0.01:10))
      | plot(.5+sin(0:0.01:10), .5+cos(0:0.01:10))
  World : sm_lib/Frames and Transforms/World Frame
  X : sm_lib/Joints/Prismatic Joint  SenseConstraintForce=off  SenseConstraintForceX=off  SenseConstraintForceY=off  SenseConstraintForceZ=off  SenseConstraintTorque=off  SenseConstraintTorqueX=off  SenseConstraintTorqueY=off  SenseConstraintTorqueZ=off  SenseTotalForce=off  SenseTotalForceX=off  SenseTotalForceY=off  SenseTotalForceZ=off  SenseTotalTorque=off  SenseTotalTorqueX=off  SenseTotalTorqueY=off  SenseTotalTorqueZ=off  CompositeWrenchDir=FollowerOnBase  CompositeWrenchFrame=BaseFrame  EquilibriumPosition=0  EquilibriumPositionUnits=m  SpringStiffness=0  SpringStiffnessUnits=N/m  DampingCoefficient=0  DampingCoefficientUnits=N/(m/s)  TorqueActuationMode=InputTorque  MotionActuationMode=ComputedMotion  SensePosition=on  SenseVelocity=on  SenseAcceleration=off  SenseTorqueForce=off  SenseLowerLimitTorqueForce=off  SenseUpperLimitTorqueForce=off  LowerLimitSpecify=off  LowerLimitBound=-1  LowerLimitBoundUnits=m  LowerLimitStiffness=1e6  LowerLimitStiffnessUnits=N/m  LowerLimitDamping=1e3  LowerLimitDampingUnits=N/(m/s)  LowerLimitTransitionRegionWidth=1e-4  LowerLimitTransitionRegionWidthUnits=m  UpperLimitSpecify=off  UpperLimitBound=1  UpperLimitBoundUnits=m  UpperLimitStiffness=1e6  UpperLimitStiffnessUnits=N/m  UpperLimitDamping=1e3  UpperLimitDampingUnits=N/(m/s)  UpperLimitTransitionRegionWidth=1e-4  UpperLimitTransitionRegionWidthUnits=m  PositionTargetSpecify=off  PositionTargetPriority=High  PositionTargetValue=0  PositionTargetValueUnits=m  VelocityTargetSpecify=off  VelocityTargetPriority=High  VelocityTargetValue=0  VelocityTargetValueUnits=m/s
  toPhi : Subsystem
  toPsi : Subsystem
  toTheta : Subsystem
  y : Outport
  wires:
  [Theta] -> Out/1(Theta)
  [Psi] -> Out/2(Psi)
  Out/1(theta) -> Mux/1  "theta"
  Out/2(psi) -> Mux/2  "psi"
  Out/3(theta_dot) -> Mux/3  "theta_dot"
  Out/4(psi_dot) -> Mux/4  "psi_dot"
  Out/5(phi) -> Mux/5  "phi"
  Out/6(phi_dot) -> Mux/6  "phi_dot"
  [Phi] -> Out/3(Phi)
  Demux/1 -> Motor_tf/2(V)
  Demux/2 -> Motor_tf2/2(V)
  V/1 -> Demux/1
  Motor_tf/2(M) -> Calc_ft/2(M_L)
  Add3/1 -> Selector/1
  [Theta] -> Add3/1
  [Psi] -> Add3/2
  Motor_tf/1(Mb) -> Calc_ft/1(Mb_L)
  Motor_tf2/1(Mb) -> Calc_ft/3(Mb_R)
  Motor_tf2/2(M) -> Calc_ft/4(M_R)
  Selector/1 -> Motor_tf/1(theta_m_dot), Motor_tf2/1(theta_m_dot), Radians to Degrees/1
  Radians to Degrees/1 -> Scope/1
  Mux/1 -> y/1
  connections:
  MechanismConfiguration/RConn1 -- Solver Configuration/RConn1 -- Psi/RConn1 -- To wheels plane/RConn1
  Rigid Transform2/LConn1 -- Wheels/LConn1 -- Rigid Transform4/LConn1
  Rigid Transform/RConn1 -- Phi/LConn1
  World/RConn1 -- Rigid Transform/LConn1
  toTheta/LConn1 -- X/RConn2
  toPhi/LConn2 -- Phi/RConn3
  toPhi/LConn1 -- Phi/RConn2
  toTheta/LConn2 -- X/RConn3
  Calc_ft/RConn1 -- Phi/LConn2
  Psi/LConn2 -- Calc_ft/RConn3
  X/LConn1 -- Rigid Transform1/RConn1
  Rigid Transform1/LConn1 -- Phi/RConn1
  Psi/RConn3 -- toPsi/LConn2
  Psi/LConn1 -- Rigid Transform4/RConn1
  X/RConn1 -- Rigid Transform2/RConn1
  X/LConn2 -- Calc_ft/RConn2
  toPsi/LConn1 -- Psi/RConn2
  To wheels plane/LConn1 -- Robot/RConn1

== system gyroboy_ext/Plant/Model/Dynamics/State-space (linear) ==
  V : Inport
  Model1 : StateSpace  A=A1  B=B1  C=C1  D=D1  InitialCondition=[0 Psi0 0 0]
  Model2 : StateSpace  A=A2  B=B2  C=C2  D=D2  InitialCondition=0
  Mux1 : Mux  Inputs=2
  y : Outport
  wires:
  Model2/1 -> Mux1/2  "y2"
  Model1/1 -> Mux1/1  "y1"
  Mux1/1 -> y/1  "y"
  V/1 -> Model2/1, Model1/1

== system gyroboy_ext/Plant/Model/Real_in/Ideal_in ==
  In : Inport
  " Out" : Outport
  wires:
  In/1 -> " Out"/1

== system gyroboy_ext/Plant/Model/Real_in/Real_in ==
  In : Inport
  Rounding Function : Rounding  Operator=round
  Saturation : Saturate  UpperLimit=100  LowerLimit=-100
  " Out" : Outport
  wires:
  In/1 -> Rounding Function/1
  Saturation/1 -> " Out"/1
  Rounding Function/1 -> Saturation/1

== system gyroboy_ext/Plant/Model/Real_out/Ideal_out ==
  "In " : Inport
  " Out" : Outport
  wires:
  "In "/1 -> " Out"/1

== system gyroboy_ext/Plant/Model/Real_out/Real_out ==
  "In " : Inport
  Rounding Function : Rounding  Operator=round
  " Out" : Outport
  wires:
  "In "/1 -> Rounding Function/1
  Rounding Function/1 -> " Out"/1

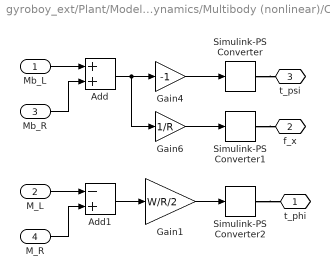
== system gyroboy_ext/Plant/Model/Dynamics/Multibody (nonlinear)/Calc_ft ==
  Mb_L : Inport
  M_L : Inport  Port=2
  Mb_R : Inport  Port=3
  M_R : Inport  Port=4
  Add : Sum
  Add1 : Sum  Inputs=-+
  Gain1 : Gain  Gain=W/R/2
  Gain4 : Gain  Gain=-1
  Gain6 : Gain  Gain=1/R
  Simulink-PS Converter : nesl_utility/Simulink-PS Converter  PhysicalDomain=network_engine_domain  SubClassName=ps_input  LeftPortType=input  RightPortType=output  PseudoPeriodic=off  Frequencies=[]  NoiseDistribution=none  NoiseParameters=[]  Unit=N*m  AffineConversion=off  FilteringAndDerivatives=zero  SimscapeFilterOrder=1  InputFilterTimeConstant=0.001  UdotUserProvided=1
  Simulink-PS Converter1 : nesl_utility/Simulink-PS Converter  PhysicalDomain=network_engine_domain  SubClassName=ps_input  LeftPortType=input  RightPortType=output  PseudoPeriodic=off  Frequencies=[]  NoiseDistribution=none  NoiseParameters=[]  Unit=N  AffineConversion=off  FilteringAndDerivatives=zero  SimscapeFilterOrder=1  InputFilterTimeConstant=0.001  UdotUserProvided=1
  Simulink-PS Converter2 : nesl_utility/Simulink-PS Converter  PhysicalDomain=network_engine_domain  SubClassName=ps_input  LeftPortType=input  RightPortType=output  PseudoPeriodic=off  Frequencies=[]  NoiseDistribution=none  NoiseParameters=[]  Unit=N*m  AffineConversion=off  FilteringAndDerivatives=zero  SimscapeFilterOrder=1  InputFilterTimeConstant=0.001  UdotUserProvided=1
  t_phi : PMIOPort  Side=Right
  f_x : PMIOPort  Port=2  Side=Right
  t_psi : PMIOPort  Port=3  Side=Right
  wires:
  Add/1 -> Gain6/1, Gain4/1
  Mb_L/1 -> Add/1
  M_L/1 -> Add1/1
  Add1/1 -> Gain1/1
  Mb_R/1 -> Add/2
  M_R/1 -> Add1/2
  Gain4/1 -> Simulink-PS Converter/1
  Gain6/1 -> Simulink-PS Converter1/1
  Gain1/1 -> Simulink-PS Converter2/1
  connections:
  Simulink-PS Converter2/RConn1 -- t_phi/RConn1
  Simulink-PS Converter/RConn1 -- t_psi/RConn1
  Simulink-PS Converter1/RConn1 -- f_x/RConn1

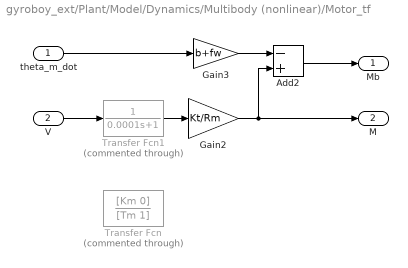
== system gyroboy_ext/Plant/Model/Dynamics/Multibody (nonlinear)/Motor_tf ==
  theta_m_dot : Inport
  V : Inport  Port=2
  Add2 : Sum  Inputs=-+
  Gain2 : Gain  Gain=Kt/Rm
  Gain3 : Gain  Gain=b+fw
  Transfer Fcn : TransferFcn  Commented=through  Numerator=[Km 0]  Denominator=[Tm 1]
  Transfer Fcn1 : TransferFcn  Commented=through  Denominator=[0.0001 1]
  Mb : Outport
  M : Outport  Port=2
  wires:
  Transfer Fcn1/1 -> Gain2/1
  Add2/1 -> Mb/1
  Gain3/1 -> Add2/1
  theta_m_dot/1 -> Gain3/1
  Gain2/1 -> M/1, Add2/2
  V/1 -> Transfer Fcn1/1

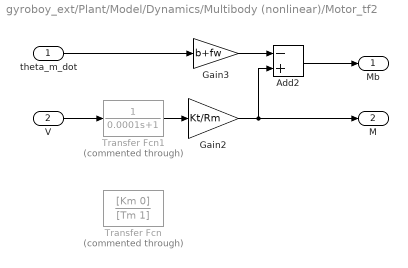
== system gyroboy_ext/Plant/Model/Dynamics/Multibody (nonlinear)/Motor_tf2 ==
  theta_m_dot : Inport
  V : Inport  Port=2
  Add2 : Sum  Inputs=-+
  Gain2 : Gain  Gain=Kt/Rm
  Gain3 : Gain  Gain=b+fw
  Transfer Fcn : TransferFcn  Commented=through  Numerator=[Km 0]  Denominator=[Tm 1]
  Transfer Fcn1 : TransferFcn  Commented=through  Denominator=[0.0001 1]
  Mb : Outport
  M : Outport  Port=2
  wires:
  Transfer Fcn1/1 -> Gain2/1
  Add2/1 -> Mb/1
  Gain3/1 -> Add2/1
  theta_m_dot/1 -> Gain3/1
  Gain2/1 -> M/1, Add2/2
  V/1 -> Transfer Fcn1/1

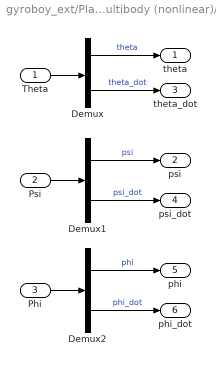
== system gyroboy_ext/Plant/Model/Dynamics/Multibody (nonlinear)/Out ==
  Theta : Inport
  Psi : Inport  Port=2
  Phi : Inport  Port=3
  Demux : Demux  Outputs=2
  Demux1 : Demux  Outputs=2
  Demux2 : Demux  Outputs=2
  theta : Outport
  psi : Outport  Port=2
  theta_dot : Outport  Port=3
  psi_dot : Outport  Port=4
  phi : Outport  Port=5
  phi_dot : Outport  Port=6
  wires:
  Psi/1 -> Demux1/1
  Theta/1 -> Demux/1
  Demux1/1 -> psi/1  "psi"
  Demux/1 -> theta/1  "theta"
  Demux1/2 -> psi_dot/1  "psi_dot"
  Demux/2 -> theta_dot/1  "theta_dot"
  Demux2/1 -> phi/1  "phi"
  Demux2/2 -> phi_dot/1  "phi_dot"
  Phi/1 -> Demux2/1

== system gyroboy_ext/Plant/Model/Dynamics/Multibody (nonlinear)/Wheels ==
  Base : sm_lib/Body Elements/Solid  InertiaType=CalculateFromGeometry  Mass=(Jw+Jm)/R^2*2  MassUnits=kg  CenterOfMass=[0 0 0]  CenterOfMassUnits=m  MomentsOfInertia=[1 1 1]  MomentsOfInertiaUnits=kg*m^2  ProductsOfInertia=[0 0 0]  ProductsOfInertiaUnits=kg*m^2  BasedOnType=Mass  Density=1000  DensityUnits=kg/(m^3)  DoExposeReferenceFrame=on  SerializedFrames=<Frames/>  GraphicType=None  MarkerShape=Sphere  MarkerSize=10  GraphicVisPropType=SimpleVisualProperties  GraphicDiffuseColor=[0.5 0.5 0.5]  GraphicSpecularColor=[0.5 0.5 0.5 1.0]  GraphicAmbientColor=[0.15 0.15 0.15 1.0]  GraphicEmissiveColor=[0.0 0.0 0.0 1.0]  GraphicShininess=75  GraphicOpacity=1.0  GeometryShape=Brick  RectangleSize=[1 1]  RectangleSizeUnits=m  BrickDimensions=[1 1 .5]*0.1  BrickDimensionUnits=m  CylinderRadius=1  CylinderRadiusUnits=m  CylinderLength=1  CylinderLengthUnits=m  SphereRadius=1  SphereRadiusUnits=m  EllipsoidRadii=[1 1 1]  EllipsoidRadiiUnits=m  ExtrusionCrossSection=[1 1; -1 1; -1 -1; 1 -1]  ExtrusionCrossSectionUnits=m  ExtrusionLength=1  ExtrusionLengthUnits=m  PolygonNumSides=3  PolygonOuterRadius=1  PolygonOuterRadiusUnits=m  ExtGeomFileType=STEP  ExtGeomFileUnits=m  RevolutionCrossSection=[1 1; 1 -1; 2 -1; 2 1]  RevolutionCrossSectionUnits=m  RevolutionExtent=Full  RevolutionAngle=180  RevolutionAngleUnits=deg
  Rigid Transform1 : sm_lib/Frames and Transforms/Rigid Transform  TranslationMethod=StandardAxis  TranslationStandardOffset=0.05  TranslationLengthUnit=m  TranslationStandardAxis=-Y  TranslationCartesianOffset=[0 0 0]  TranslationROffset=0  TranslationROffsetUnits=m  TranslationZOffset=0  TranslationZOffsetUnits=m  TranslationThetaOffset=0  TranslationThetaOffsetUnits=deg  RotationMethod=StandardAxis  RotationAngleUnits=deg  RotationStandardAxis=+X  RotationAngle=90  RotationArbitraryAxis=[0 0 1]  FollAlignAxisA=+X  BaseAlignAxisA=+Y  FollAlignAxisB=+Y  BaseAlignAxisB=+Z  RotationSequenceAxes=FollowerAxes  RotationSequence=XYX  RotationSequenceAngles=[0 0 0]  RotationSequenceAnglesUnits=deg  RotationMatrix=[1 0 0; 0 1 0; 0 0 1]
  Rigid Transform3 : sm_lib/Frames and Transforms/Rigid Transform  TranslationMethod=StandardAxis  TranslationStandardOffset=0.05  TranslationLengthUnit=m  TranslationStandardAxis=+Y  TranslationCartesianOffset=[0 0 0]  TranslationROffset=0  TranslationROffsetUnits=m  TranslationZOffset=0  TranslationZOffsetUnits=m  TranslationThetaOffset=0  TranslationThetaOffsetUnits=deg  RotationMethod=StandardAxis  RotationAngleUnits=deg  RotationStandardAxis=+X  RotationAngle=90  RotationArbitraryAxis=[0 0 1]  FollAlignAxisA=+X  BaseAlignAxisA=+Y  FollAlignAxisB=+Y  BaseAlignAxisB=+Z  RotationSequenceAxes=FollowerAxes  RotationSequence=XYX  RotationSequenceAngles=[0 0 0]  RotationSequenceAnglesUnits=deg  RotationMatrix=[1 0 0; 0 1 0; 0 0 1]
  Wheel1 : sm_lib/Body Elements/Solid  InertiaType=PointMass  Mass=0  MassUnits=g  CenterOfMass=[0 0 0]  CenterOfMassUnits=m  MomentsOfInertia=[0 0 0]  MomentsOfInertiaUnits=kg*m^2  ProductsOfInertia=[0 0 0]  ProductsOfInertiaUnits=kg*m^2  BasedOnType=Mass  Density=1000  DensityUnits=kg/(m^3)  DoExposeReferenceFrame=on  SerializedFrames=<Frames/>  GraphicType=FromGeometry  MarkerShape=Sphere  MarkerSize=10  GraphicVisPropType=SimpleVisualProperties  GraphicDiffuseColor=[1.0 0.4 0.4]  GraphicSpecularColor=[0.5 0.5 0.5 1.0]  GraphicAmbientColor=[0.15 0.15 0.15 1.0]  GraphicEmissiveColor=[0.0 0.0 0.0 1.0]  GraphicShininess=75  GraphicOpacity=1.0  GeometryShape=Cylinder  RectangleSize=[1 1]  RectangleSizeUnits=m  BrickDimensions=[1 1 1]  BrickDimensionUnits=m  CylinderRadius=R  CylinderRadiusUnits=m  CylinderLength=0.02  CylinderLengthUnits=m  SphereRadius=1  SphereRadiusUnits=m  EllipsoidRadii=[1 1 1]  EllipsoidRadiiUnits=m  ExtrusionCrossSection=[1 1; -1 1; -1 -1; 1 -1]  ExtrusionCrossSectionUnits=m  ExtrusionLength=1  ExtrusionLengthUnits=m  PolygonNumSides=3  PolygonOuterRadius=1  PolygonOuterRadiusUnits=m  ExtGeomFileType=STEP  ExtGeomFileUnits=m  RevolutionCrossSection=[1 1; 1 -1; 2 -1; 2 1]  RevolutionCrossSectionUnits=m  RevolutionExtent=Full  RevolutionAngle=180  RevolutionAngleUnits=deg
  Wheel2 : sm_lib/Body Elements/Solid  InertiaType=PointMass  Mass=0  MassUnits=g  CenterOfMass=[0 0 0]  CenterOfMassUnits=m  MomentsOfInertia=[0 0 0]  MomentsOfInertiaUnits=kg*m^2  ProductsOfInertia=[0 0 0]  ProductsOfInertiaUnits=kg*m^2  BasedOnType=Mass  Density=1000  DensityUnits=kg/(m^3)  DoExposeReferenceFrame=on  SerializedFrames=<Frames/>  GraphicType=FromGeometry  MarkerShape=Sphere  MarkerSize=10  GraphicVisPropType=SimpleVisualProperties  GraphicDiffuseColor=[1.0 0.4 0.4]  GraphicSpecularColor=[0.5 0.5 0.5 1.0]  GraphicAmbientColor=[0.15 0.15 0.15 1.0]  GraphicEmissiveColor=[0.0 0.0 0.0 1.0]  GraphicShininess=75  GraphicOpacity=1.0  GeometryShape=Cylinder  RectangleSize=[1 1]  RectangleSizeUnits=m  BrickDimensions=[1 1 1]  BrickDimensionUnits=m  CylinderRadius=R  CylinderRadiusUnits=m  CylinderLength=0.02  CylinderLengthUnits=m  SphereRadius=1  SphereRadiusUnits=m  EllipsoidRadii=[1 1 1]  EllipsoidRadiiUnits=m  ExtrusionCrossSection=[1 1; -1 1; -1 -1; 1 -1]  ExtrusionCrossSectionUnits=m  ExtrusionLength=1  ExtrusionLengthUnits=m  PolygonNumSides=3  PolygonOuterRadius=1  PolygonOuterRadiusUnits=m  ExtGeomFileType=STEP  ExtGeomFileUnits=m  RevolutionCrossSection=[1 1; 1 -1; 2 -1; 2 1]  RevolutionCrossSectionUnits=m  RevolutionExtent=Full  RevolutionAngle=180  RevolutionAngleUnits=deg
  B : PMIOPort  Side=Left
  connections:
  Wheel2/RConn1 -- Rigid Transform3/RConn1
  Wheel1/RConn1 -- Rigid Transform1/RConn1
  Rigid Transform1/LConn1 -- Base/RConn1 -- Rigid Transform3/LConn1 -- B/RConn1

== system gyroboy_ext/Plant/Model/Dynamics/Multibody (nonlinear)/toPhi ==
  Mux : Mux  Inputs=2
  PS-Simulink Converter : nesl_utility/PS-Simulink Converter  PhysicalDomain=network_engine_domain  SubClassName=ps_output  LeftPortType=input  RightPortType=output  PseudoPeriodic=off  Frequencies=[]  Unit=rad  AffineConversion=off
  PS-Simulink Converter1 : nesl_utility/PS-Simulink Converter  PhysicalDomain=network_engine_domain  SubClassName=ps_output  LeftPortType=input  RightPortType=output  PseudoPeriodic=off  Frequencies=[]  Unit=rad/s  AffineConversion=off
  q : PMIOPort  Side=Left
  w : PMIOPort  Port=2  Side=Left
  tag scope: Phi=global
  wires:
  PS-Simulink Converter/1 -> Mux/1
  PS-Simulink Converter1/1 -> Mux/2
  Mux/1 -> [Phi]
  connections:
  PS-Simulink Converter/LConn1 -- q/RConn1
  PS-Simulink Converter1/LConn1 -- w/RConn1

== system gyroboy_ext/Plant/Model/Dynamics/Multibody (nonlinear)/toPsi ==
  Mux : Mux  Inputs=2
  PS-Simulink Converter : nesl_utility/PS-Simulink Converter  PhysicalDomain=network_engine_domain  SubClassName=ps_output  LeftPortType=input  RightPortType=output  PseudoPeriodic=off  Frequencies=[]  Unit=rad  AffineConversion=off
  PS-Simulink Converter1 : nesl_utility/PS-Simulink Converter  PhysicalDomain=network_engine_domain  SubClassName=ps_output  LeftPortType=input  RightPortType=output  PseudoPeriodic=off  Frequencies=[]  Unit=rad/s  AffineConversion=off
  q : PMIOPort  Side=Left
  w : PMIOPort  Port=2  Side=Left
  tag scope: Psi=global
  wires:
  PS-Simulink Converter1/1 -> Mux/2
  Mux/1 -> [Psi]
  PS-Simulink Converter/1 -> Mux/1
  connections:
  PS-Simulink Converter/LConn1 -- q/RConn1
  PS-Simulink Converter1/LConn1 -- w/RConn1

== system gyroboy_ext/Plant/Model/Dynamics/Multibody (nonlinear)/toTheta ==
  Gain : Gain  Gain=1/R
  Mux : Mux  Inputs=2
  PS-Simulink Converter : nesl_utility/PS-Simulink Converter  PhysicalDomain=network_engine_domain  SubClassName=ps_output  LeftPortType=input  RightPortType=output  PseudoPeriodic=off  Frequencies=[]  Unit=m  AffineConversion=off
  PS-Simulink Converter1 : nesl_utility/PS-Simulink Converter  PhysicalDomain=network_engine_domain  SubClassName=ps_output  LeftPortType=input  RightPortType=output  PseudoPeriodic=off  Frequencies=[]  Unit=m/s  AffineConversion=off
  px : PMIOPort  Side=Left
  vx : PMIOPort  Port=2  Side=Left
  tag scope: Theta=global
  wires:
  PS-Simulink Converter1/1 -> Mux/2
  Gain/1 -> [Theta]
  Mux/1 -> Gain/1
  PS-Simulink Converter/1 -> Mux/1
  connections:
  PS-Simulink Converter/LConn1 -- px/RConn1
  PS-Simulink Converter1/LConn1 -- vx/RConn1

== stateflow chart gyroboy_ext/Controller/PWM Control ==
  state On
    entry:
    MODE = 1;
    state OK = check(PWM) [function]
    state Normal
    state Emergency
    (default) -> Normal
    Normal -> Emergency : [~check(PWM)]
    Emergency -> Normal [order 1] : [check(PWM)]
  state Off
    entry:
    MODE = 0;
  (default) -> On
  Emergency -> Off [order 2] : after(0.5,sec)
  Off -> On : [Data.btn]
  data: PWM function_input double size=2; OK function_output size=1; PWM input; MODE output =1; Data input Bus: Data

== matlab function gyroboy_ext/Plant/Model/get sensors ==
  data: enc_l output; enc_r output; y input; gyro output; R parameter; W parameter
function [enc_l, enc_r, gyro] = sensors(y, R, W)
enc_l = rad2deg(y(1) - W/R/2 * y(5) - y(2));
enc_r = rad2deg(y(1) + W/R/2 * y(5) - y(2));
gyro  = rad2deg(y(4));

== matlab function gyroboy_ext/Controller/SET COLOR ==
  data: M input; C output
function C = fcn(M)
switch M
    case 0
        C = 2; % Red if Emergency off
    case 1
        C = 1; % Green if Running
    otherwise
        C = 0; % No light
end

== stateflow chart gyroboy_ext/Controller/Distance Control ==
  state Normal
  state STOP
  (default) -> Normal
  Normal -> STOP : [Data.usonic < 10]
  STOP -> Normal : [Data.usonic > 15]
  data: sf_internal_action_state_placeholder_data local double size=1 =0; sf_internal_action_state_placeholder_data local double size=1 =0; Data input Bus: Data; ref output size=2
